simulink model "dsppitchtime"  (Simulink 6.0)
settings: Solver=FixedStepDiscrete  StartTime=0.0  StopTime=4  RelTol=1e-3
PreLoadFcn:
  | load clean_speech.mat;
values from neighbouring files (symbols this model uses):
  D = var(Noisef)    [lmsxy.m]
libraries: dspsigops x5, dspmtrx3 x4, dspobslib x4, dspsrcs4 x2, dspxfrm3 x2, dspsigattribs x1, simulink x1, dspbuff3 x1, dspswit3 x1, dspsnks4 x1
CloseFcn:
  | clear Fs Fs_new Speech Ts ahop blk blk2 shop y_pnt
settings Model: Creator=mkhan  LastModifiedBy=mkhan  ExtModeAutoUpdateStatusClock=off  ProdHWDeviceType=Specified
settings DataIOCC: LimitDataPoints=off  SaveTime=off  OutputSaveName=y_pnt  SignalLoggingName=logsOut
settings OptimizationCC: InlineParams=on
settings DebuggingCC: CheckExecutionContextPreStartOutputMsg=on  CheckExecutionContextRuntimeOutputMsg=on  SolverPrmCheckMsg=none
settings HardwareCC: ProdHWDeviceType=Specified
settings SFSimCC: SFSimApplyToAllLibs=on  SFSimBuildMode=Incremental

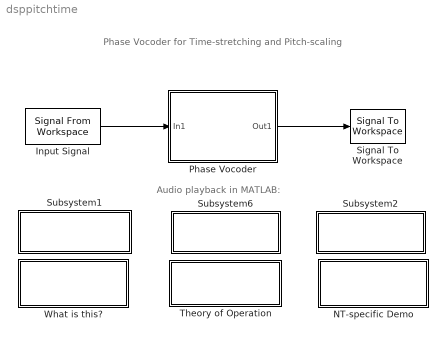
== system dsppitchtime ==
  note: Audio playback in MATLAB:
  note: Phase Vocoder for Time-stretching and Pitch-scaling
  Input Signal : dspsrcs4/Signal From Workspace  X=Speech  Ts=1/8000  nsamps=64  OutputAfterFinalValue=Setting to zero
  NT-specific Demo : Subsystem  PropExecContextAcrossSSBoundary=on
      settings: OpenFcn=dsppitchtime_win32
      mask Type: NT-only Demo
      mask Display: disp('PC/Windows\nDemo')
  Phase Vocoder : Subsystem  PropExecContextAcrossSSBoundary=on  mask(Phase Vocoder){ana_hopSize=64, winLen=256, syn_hopSize=90}
      mask prompts: ana_hopSize "Analysis hop-size (i.e., temporal shift of analysis window) (in samples):"; winLen "Window size (in samples):"; syn_hopSize "Synthesis hop-size (i.e., temporal shift of synthesis window) (in samples):"
      mask help:
      | Algorithm for time-stretching and pitch-scaling of an audio signal. Time-stretching changes the speed of an audio signal without affecting its pitch. Pitch-scaling changes the pitch of an audio signal without affecting its speed.
      |
      | The pitch-scaling and time-stretching factors are defined by the ratio of the Synthesis hop-size parameter to the Analysis hop-size parameter.
      |
      | The Window size parameter must meet the following two requirements:
      | - log2(Window size) must be a positive integer
      | - Window size must be greater than both the Analysis hop-size and the Synthesis hop-size parameter values.
      mask Display: disp('Phase Vocoder')
  Signal To Workspace : dspsnks4/Signal To Workspace  VariableName=y_pnt  FrameMode=Concatenate frames (2-D array)
      settings: FixptAsFi=off
  Subsystem1 : Subsystem  PropExecContextAcrossSSBoundary=on
      settings: OpenFcn=|
      | blk = 'dsppitchtime/Input Signal';
      | Ts = get_param(blk,'Ts');
      | Fs = 1/str2num(Ts);
      | if exist('Speech','var'), soundsc(Speech(200:end),Fs); else uiwait(errordlg('Data not found in workspace - reload demo model.','Signal Processing Blockset Demo Error','modal'));end
      mask Display: disp('Original\nSignal')
  Subsystem2 : Subsystem  PropExecContextAcrossSSBoundary=on
      settings: OpenFcn=|
      | blk = 'dsppitchtime/Input Signal';
      | Ts = get_param(blk,'Ts');
      | Fs = 1/str2num(Ts);
      | 
      | if exist('y_pnt','var'), soundsc(y_pnt(200:end),Fs); else uiwait(errordlg('You must run the simulation first.','Signal Processing Blockset Demo Error','modal')); end
      mask Display: disp('Time-stretched\nSignal')
  Subsystem6 : Subsystem  StopFcn=|  PropExecContextAcrossSSBoundary=on
      | blk = 'dsppitchtime/Input Signal';                                                                          
      | Ts = get_param(blk,'Ts');                                                                                   
      | Fs = 1/str2num(Ts);                                                                                         
      | blk2 = 'dsppitchtime/Phase Vocoder';                                                                        
      | ahop =str2num(get_param(blk2,'ana_hopSize'));                                                               
      | shop =str2num(get_param(blk2,'syn_hopSize'));                                                               
      | Fs_new = Fs*(shop/ahop);                                                                                    
      | if exist('y_pnt','var'),                                                                                    
      |     soundsc(y_pnt(200:end),Fs_new);                                                                         
      | else uiwait(errordlg('You must run the simulation first.','Signal Processing Blockset Demo Error','modal'));
      | end
      settings: OpenFcn=|
      | blk = 'dsppitchtime/Input Signal';
      | Ts = get_param(blk,'Ts');
      | Fs = 1/str2num(Ts);
      | blk2 = 'dsppitchtime/Phase Vocoder';
      | ahop =str2num(get_param(blk2,'ana_hopSize'));
      | shop =str2num(get_param(blk2,'syn_hopSize'));
      | Fs_new = Fs*(shop/ahop);
      | if exist('y_pnt','var'),
      |     soundsc(y_pnt(200:end),Fs_new);
      | else uiwait(errordlg('You must run the simulation first.','Signal Processing Blockset Demo Error','modal'));
      | end
      mask Display: disp('Pitch-scaled\nSignal')
  Theory of Operation : Subsystem  PropExecContextAcrossSSBoundary=on
      mask Type: Theory of Operation
      mask Display: disp('Theory of\nOperation')
  What is this? : Subsystem  PropExecContextAcrossSSBoundary=on
      mask Type: Frame-Based Simulation Info
      mask Display: disp('What is this?')
  wires:
  Phase Vocoder/1(Out1) -> Signal To Workspace/1
  Input Signal/1 -> Phase Vocoder/1(In1)

== system dsppitchtime/NT-specific Demo ==

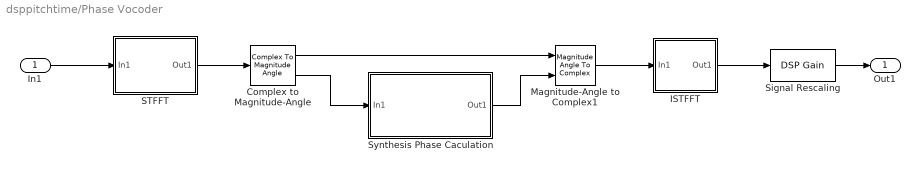
== system dsppitchtime/Phase Vocoder ==
  In1 : Inport  LatchInput=off
  Complex to Magnitude-Angle : ComplexToMagnitudeAngle
  ISTFFT : Subsystem  PropExecContextAcrossSSBoundary=on
      mask Display: disp('Overlap\nIST-FFT')
  Magnitude-Angle to Complex1 : MagnitudeAngleToComplex
  STFFT : Subsystem  PropExecContextAcrossSSBoundary=on
      mask Display: disp('Overlap\nST-FFT')
  Signal Rescaling : dspobslib/DSP Gain  gainValue=1/(winLen*sum(hanning(winLen,'periodic').^2)/syn_hopSize)  roundingMode=Floor  overflowMode=off
  Synthesis Phase Caculation : Subsystem  PropExecContextAcrossSSBoundary=on  mask{ana_hopSize=ana_hopSize, syn_hopSize=syn_hopSize, winLen=winLen}
      mask prompts: ana_hopSize "Analysis hop size:"; syn_hopSize "Synthesis hop size:"; winLen "Window size:"
      mask Display: disp('Synthesis\nPhase\nCalculation')
  Out1 : Outport
  wires:
  In1/1 -> STFFT/1(In1)
  STFFT/1(Out1) -> Complex to Magnitude-Angle/1
  Magnitude-Angle to Complex1/1 -> ISTFFT/1(In1)
  ISTFFT/1(Out1) -> Signal Rescaling/1
  Complex to Magnitude-Angle/2 -> Synthesis Phase Caculation/1(In1)
  Complex to Magnitude-Angle/1 -> Magnitude-Angle to Complex1/1
  Synthesis Phase Caculation/1(Out1) -> Magnitude-Angle to Complex1/2
  Signal Rescaling/1 -> Out1/1

== system dsppitchtime/Subsystem1 ==

== system dsppitchtime/Subsystem2 ==

== system dsppitchtime/Subsystem6 ==

== system dsppitchtime/Theory of Operation ==
  note: This simulation demonstrates time-stretching or pitch-scaling effect
      | applied to audio signal using Phase Vocoder. To see the
      | implementation "Look Under" the "Phase Vocoder" block by selecting
      | the block and either hitting "ctrl+u", or right clicking on the block and
      | selecting "Look Under Mask."
      |
      | For further information you may also refer to the following paper:
      | A. D. Gotzen, N. Bernardini and D. Arfib, "Traditional Implementations
      | of a Phase-Vocoder: The Tricks of the Trade," Proc. of the COST G-6
      | Conference on Digital Audio Effects (DAFX-00), Verona, Italy,
      | December 7-9, 2000.

== system dsppitchtime/What is this? ==
  note: This simulation demonstrates how to use a phase vocoder to
      | implement time-stretching and pitch-scaling of an audio signal.
      |
      | Run the simulation. The pitch-scaled signal is automatically played
      | once the simulation has finished. To play the Original Signal,
      | double-click the block labeled "Original Signal". To play
      | the Pitch-scaled Signal or the Time-stretched Signal, double-click
      | the blocks labeled "Pitch-scaled Signal" or "Time-stretched Signal".
      |
      | Double-click the Phase Vocoder block. Change the Synthesis hop-size
      | parameter to 64, the same value as the Analysis hop-size parameter.
      | Run the simulation and listen to the three signals. The Pitch-scaled
      | Signal has the same pitch as the Original Signal, and the Time-stretched
      | Signal has the same speed as the Original Signal.
      |
      | Double-click the Phase Vocoder block. Change the Synthesis hop-size
      | parameter to 48, which is less than the Analysis hop-size parameter.
      | Run the simulation and listen to the three signals. The Pitch-scaled
      | Signal has a lower pitch than the Original Signal. The Time-stretched
      | Signal is faster than the Original Signal.

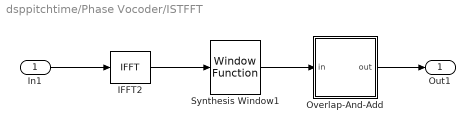
== system dsppitchtime/Phase Vocoder/ISTFFT ==
  In1 : Inport  LatchInput=off
  IFFT2 : dspxfrm3/IFFT  DialogController=dspDDGCreate  DialogControllerArgs=DataTag0  CompMethod=Table lookup  TableOpt=Speed  BitRevOrder=off  cs_in=on  SkipNorm=on  mode=Complex  firstCoeffMode=User-defined  firstCoeffWordLength=16  firstCoeffFracLength=15  roundingMode=Floor  overflowMode=off
  Overlap-And-Add : Subsystem  PropExecContextAcrossSSBoundary=on  mask(Overlap-And-Add){L=syn_hopSize}
      mask prompts: L "Number of new points in each frame"
      mask help: Performs overlap-and-add on the input signal. Disjoint frames of the input signal are overlapped with each other for a specified number of points and summed.
      mask Display: disp('Overlap\nAnd\nAdd')
  Synthesis Window1 : dspsigops/Window Function  DialogController=dspDDGCreate  DialogControllerArgs=DataTag1  winmode=Apply window to input  wintype=Hanning  sampmode=Continuous  samptime=1  N=64  Rs=50  beta=10  winsamp=Periodic  UserWindow=hamming  OptParams=off  UserParams={1.0}  dataType=double  isSigned=on  wordLen=16  udDataType=sfix(16)  fracBitsMode=Best precision  numFracBits=15  roundingMode=Floor  overflowMode=off
  Out1 : Outport
  wires:
  IFFT2/1 -> Synthesis Window1/1
  Overlap-And-Add/1(out) -> Out1/1
  In1/1 -> IFFT2/1
  Synthesis Window1/1 -> Overlap-And-Add/1(in)

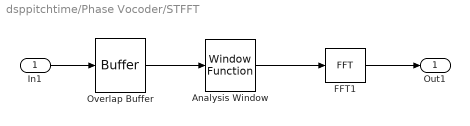
== system dsppitchtime/Phase Vocoder/STFFT ==
  In1 : Inport  LatchInput=off
  Analysis Window : dspsigops/Window Function  DialogController=dspDDGCreate  DialogControllerArgs=DataTag2  winmode=Apply window to input  wintype=Hanning  sampmode=Continuous  samptime=1  N=64  Rs=50  beta=10  winsamp=Periodic  UserWindow=hamming  OptParams=off  UserParams={1.0}  dataType=double  isSigned=on  wordLen=16  udDataType=sfix(16)  fracBitsMode=Best precision  numFracBits=15  roundingMode=Floor  overflowMode=off
  FFT1 : dspxfrm3/FFT  DialogController=dspDDGCreate  DialogControllerArgs=DataTag3  CompMethod=Table lookup  TableOpt=Speed  BitRevOrder=off  SkipNorm=off  firstCoeffMode=User-defined  firstCoeffWordLength=16  firstCoeffFracLength=15  roundingMode=Floor  overflowMode=off
  Overlap Buffer : dspbuff3/Buffer  N=winLen  V=winLen-ana_hopSize  ic=0
  Out1 : Outport
  wires:
  Overlap Buffer/1 -> Analysis Window/1
  FFT1/1 -> Out1/1
  In1/1 -> Overlap Buffer/1
  Analysis Window/1 -> FFT1/1

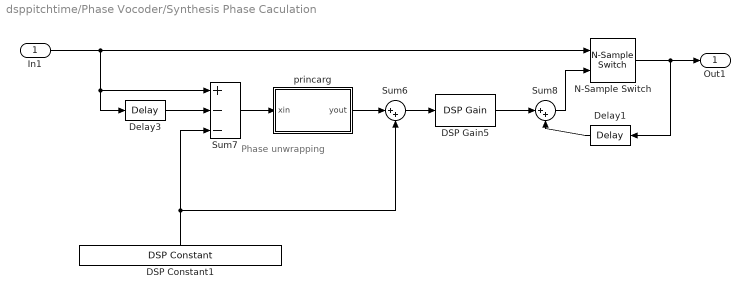
== system dsppitchtime/Phase Vocoder/Synthesis Phase Caculation ==
  note: Phase unwrapping
  In1 : Inport  LatchInput=off
  DSP Constant1 : dspsrcs4/DSP Constant  Orientation=up  Value=2*pi*ana_hopSize*[0:winLen-1]'/winLen  SampleMode=Discrete  discreteOutput=Sample-based  continuousOutput=Sample-based  sampTime=64/8000  framePeriod=2  dataType=Inherit from 'Constant value'  isSigned=on  wordLen=16  udDataType=sfix(16)  fracBitsMode=Best precision  numFracBits=15  InterpretAs1D=-inf  Ts=-inf  FramebasedOutput=-inf
  DSP Gain5 : dspobslib/DSP Gain  gainValue=syn_hopSize/ana_hopSize  roundingMode=Floor  overflowMode=off
  Delay1 : dspsigops/Delay  Orientation=left  dly_unit=Frames  delay=1  ic_detail=on  dif_ic_for_ch=off  dif_ic_for_dly=off  ic=0  reset_popup=None
  Delay3 : dspsigops/Delay  dly_unit=Frames  delay=1  ic_detail=on  dif_ic_for_ch=off  dif_ic_for_dly=off  ic=0  reset_popup=None
  N-Sample Switch : dspswit3/N-Sample Switch  N=1  reset=off  TriggerType=Rising edge  Ts=-1
  Sum6 : Sum  Inputs=|++  SaturateOnIntegerOverflow=on
  Sum7 : Sum  Inputs=+--  SaturateOnIntegerOverflow=on
  Sum8 : Sum  Inputs=|++  SaturateOnIntegerOverflow=on
  princarg : Subsystem  PropExecContextAcrossSSBoundary=on
      mask Display: disp('Principal\nArgument');
  Out1 : Outport
  wires:
  In1/1 -> N-Sample Switch/1, Delay3/1, Sum7/1
  Delay3/1 -> Sum7/2
  DSP Constant1/1 -> Sum7/3, Sum6/2
  Sum7/1 -> princarg/1(xin)
  princarg/1(yout) -> Sum6/1
  Sum6/1 -> DSP Gain5/1
  DSP Gain5/1 -> Sum8/1
  N-Sample Switch/1 -> Delay1/1, Out1/1
  Delay1/1 -> Sum8/2
  Sum8/1 -> N-Sample Switch/2

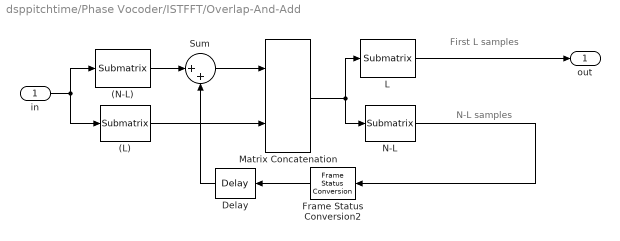
== system dsppitchtime/Phase Vocoder/ISTFFT/Overlap-And-Add ==
  note: First L samples
  note: N-L samples
  in : Inport  LatchInput=off
  (L) : dspmtrx3/Submatrix  RowSpan=Range of rows  RowStartMode=Offset from last  RowStartIndex=L-1  RowEndMode=Last  RowEndIndex=1  ColSpan=All columns  ColStartMode=First  ColStartIndex=1  ColEndMode=Last  ColEndIndex=1
  (N-L) : dspmtrx3/Submatrix  RowSpan=Range of rows  RowStartMode=First  RowStartIndex=1  RowEndMode=Offset from last  RowEndIndex=L  ColSpan=All columns  ColStartMode=First  ColStartIndex=1  ColEndMode=Last  ColEndIndex=1
  Delay : dspsigops/Delay  Orientation=left  dly_unit=Samples  delay=1  ic_detail=off  dif_ic_for_ch=off  dif_ic_for_dly=off  ic=0  reset_popup=None
  Frame Status Conversion2 : dspsigattribs/Frame Status Conversion  Orientation=left  growRefPort=off  outframe=Sample-based
  L : dspmtrx3/Submatrix  RowSpan=Range of rows  RowStartMode=First  RowStartIndex=1  RowEndMode=Index  RowEndIndex=L  ColSpan=All columns  ColStartMode=First  ColStartIndex=1  ColEndMode=Last  ColEndIndex=1
  Matrix Concatenation : simulink/Math Operations/Matrix Concatenation  numInports=2  catMethod=Vertical
  N-L : dspmtrx3/Submatrix  RowSpan=Range of rows  RowStartMode=Index  RowStartIndex=L+1  RowEndMode=Last  RowEndIndex=1  ColSpan=All columns  ColStartMode=First  ColStartIndex=1  ColEndMode=Last  ColEndIndex=1
  Sum : Sum  Inputs=|++  SaturateOnIntegerOverflow=on  InputSameDT=on
  out : Outport
  wires:
  L/1 -> out/1
  Sum/1 -> Matrix Concatenation/1
  (N-L)/1 -> Sum/1
  Delay/1 -> Sum/2
  (L)/1 -> Matrix Concatenation/2
  N-L/1 -> Frame Status Conversion2/1
  Matrix Concatenation/1 -> L/1, N-L/1
  in/1 -> (L)/1, (N-L)/1
  Frame Status Conversion2/1 -> Delay/1

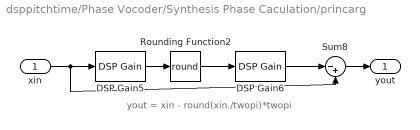
== system dsppitchtime/Phase Vocoder/Synthesis Phase Caculation/princarg ==
  note: yout = xin - round(xin./twopi)*twopi
  xin : Inport  LatchInput=off
  DSP Gain5 : dspobslib/DSP Gain  gainValue=1/(2*pi)  roundingMode=Floor  overflowMode=off
  DSP Gain6 : dspobslib/DSP Gain  gainValue=2*pi  roundingMode=Floor  overflowMode=off
  Rounding Function2 : Rounding  Operator=round
  Sum8 : Sum  Inputs=|-+  SaturateOnIntegerOverflow=on
  yout : Outport
  wires:
  xin/1 -> Sum8/2, DSP Gain5/1
  DSP Gain5/1 -> Rounding Function2/1
  Rounding Function2/1 -> DSP Gain6/1
  DSP Gain6/1 -> Sum8/1
  Sum8/1 -> yout/1
